simulink model "MSFartoystyring"  (R2013a)
settings: Solver=ode45  StartTime=tstart  StopTime=tstop  RelTol=1e-3
values from neighbouring files (symbols this model uses):
  c = 1    [run.m]
  K_d = (20*xsi*omega_n*T-1)/K    [run.m]
  K_i = 0    [run.m]
  K_i2 = 0.005    [run.m]
  K_p = ((omega_n^2)*T)/K    [run.m]
  K_p2 = 20    [run.m]
  psi0 = 0    [run.m]
  psi_desired = deg2rad(90)    [run.m]
  r0 = 0    [run.m]
  tsamp = 10    [run.m]
  u_desired = 7.3    [run.m]
  v0 = [0.1 0]'    [run.m]
undefined symbols (not defined in the file or in its folder): msfartoystyring
undefined symbols (not defined in the file): p0
settings Model: ExtModeAutoUpdateStatusClock=off  Creator=christh  LastModifiedBy=Mat
settings DataIOCC: SignalLoggingSaveFormat=ModelDataLogs
settings OptimizationCC: ExpressionDepthLimit=2147483647  InitFltsAndDblsToZero=on
settings DebuggingCC: FcnCallInpInsideContextMsg=UseLocalSettings
settings GRTTargetCC: CombineOutputUpdateFcns=off  GRTInterface=on

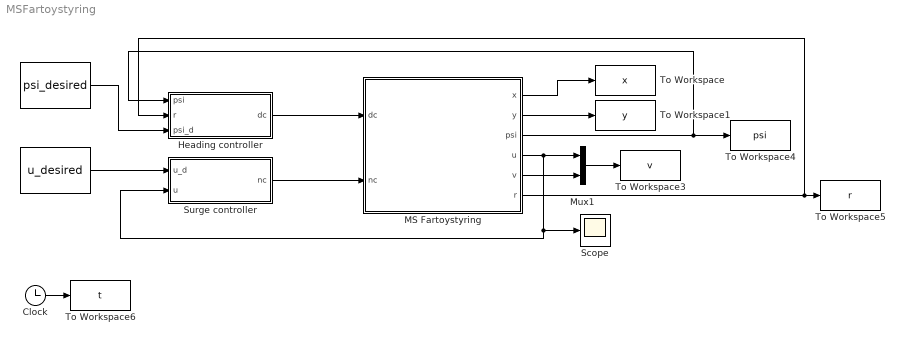
== system MSFartoystyring ==
  " " : Constant  Value=psi_desired
  " " : Constant  Value=u_desired
  Clock : Clock
  Heading controller : Subsystem
  MS Fartoystyring : Subsystem  mask(MS Fartoystyring for Assignment 3 G&C){x0=p0(1), y0=p0(2), u0=v0(1), v0=v0(2), psi0=psi0, r0=r0, c=c}
      mask prompts: x0 "x(t0) (m)"; y0 "y(t0) (m)"; u0 "u(t0) (m/s)"; v0 "v(t0) (m/s)"; psi0 "psi(t0) (rad)"; r0 "r(t0) (rad/s)"; c "current (0 or 1)"
      mask help:
      | Block corresponding to Figure 1 in the assignment text. Gives the response of the ship.
      |
      | The design speed of MS Fartoystyring is u=8.23 m/s.
      |
      | Input:
      | dc: commanded rudder (rad), dmax=25*pi/180
      | nc: commanded shaft speed (rad/s), nmax=85*2*pi/60
      |
      | Output:
      | x: north pos (m)
      | y: east pos (m)
      | u: surge (m/s)
      | v: sway (m/s)
      | psi: heading (rad)
      | r: yaw (rad/s)
      mask Help: Comments, bugs and help requests can be directed to the TA. Email on course website.
  Mux1 : Mux  Inputs=2
  Scope : Scope
  Surge controller : Subsystem
  To Workspace : ToWorkspace  VariableName=x  SampleTime=tsamp
  To Workspace1 : ToWorkspace  VariableName=y  SampleTime=tsamp
  To Workspace3 : ToWorkspace  VariableName=v  SampleTime=tsamp
  To Workspace4 : ToWorkspace  VariableName=psi  SampleTime=tsamp
  To Workspace5 : ToWorkspace  VariableName=r  SampleTime=tsamp
  To Workspace6 : ToWorkspace  VariableName=t  SampleTime=tsamp
  wires:
  Clock/1 -> To Workspace6/1
  MS Fartoystyring/1(x) -> To Workspace/1
  MS Fartoystyring/2(y) -> To Workspace1/1
  MS Fartoystyring/5(v) -> Mux1/2
  Mux1/1 -> To Workspace3/1
  MS Fartoystyring/3(psi) -> To Workspace4/1, Heading controller/1("psi ")
  MS Fartoystyring/6(r) -> Heading controller/2(r), To Workspace5/1
  MS Fartoystyring/4(u) -> Surge controller/2("u "), Scope/1, Mux1/1
  Surge controller/1("nc ") -> MS Fartoystyring/2(nc)
  " "/1 -> Surge controller/1(u_d)
  Heading controller/1("dc ") -> MS Fartoystyring/1(dc)
  " "/1 -> Heading controller/3(psi_d)

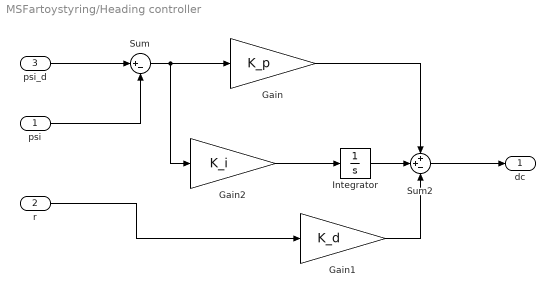
== system MSFartoystyring/Heading controller ==
  "psi " : Inport
  r : Inport  Port=2
  psi_d : Inport  Port=3
  Gain : Gain  Gain=K_p
  Gain1 : Gain  Gain=K_d
  Gain2 : Gain  Gain=K_i
  Integrator : Integrator
  Sum : Sum  Inputs=|+-
  Sum2 : Sum  Inputs=++-
  "dc " : Outport
  wires:
  psi_d/1 -> Sum/1
  "psi "/1 -> Sum/2
  Sum/1 -> Gain2/1, Gain/1
  Gain/1 -> Sum2/1
  Gain2/1 -> Integrator/1
  Integrator/1 -> Sum2/2
  r/1 -> Gain1/1
  Gain1/1 -> Sum2/3
  Sum2/1 -> "dc "/1

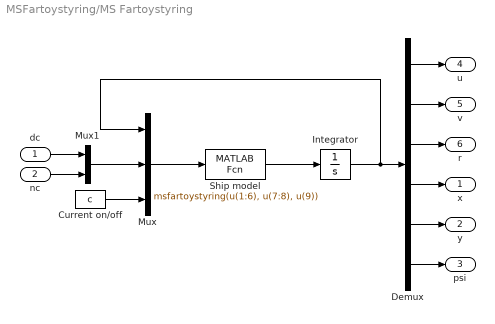
== system MSFartoystyring/MS Fartoystyring ==
  dc : Inport
  nc : Inport  Port=2
  Current on/off : Constant  Value=c
  Demux : Demux  Outputs=6
  Integrator : Integrator  InitialCondition=[u0 v0 r0 x0 y0 psi0]'
  Mux : Mux  Inputs=3
  Mux1 : Mux  Inputs=2
  Ship model : MATLABFcn  MATLABFcn=msfartoystyring(u(1:6), u(7:8), u(9))  OutputDimensions=6
  x : Outport
  y : Outport  Port=2
  psi : Outport  Port=3
  u : Outport  Port=4
  v : Outport  Port=5
  r : Outport  Port=6
  wires:
  Integrator/1 -> Mux/1, Demux/1
  Mux1/1 -> Mux/2
  dc/1 -> Mux1/1
  nc/1 -> Mux1/2
  Demux/1 -> u/1
  Demux/2 -> v/1
  Demux/3 -> r/1
  Demux/4 -> x/1
  Demux/5 -> y/1
  Demux/6 -> psi/1
  Current on/off/1 -> Mux/3
  Ship model/1 -> Integrator/1
  Mux/1 -> Ship model/1

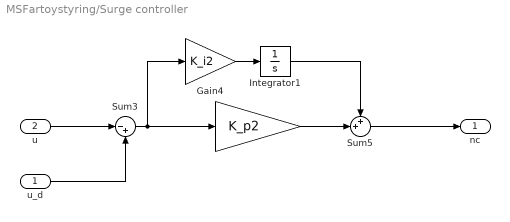
== system MSFartoystyring/Surge controller ==
  u_d : Inport
  "u " : Inport  Port=2
  " " : Gain  Gain=K_p2
  Gain4 : Gain  Gain=K_i2
  Integrator1 : Integrator
  Sum3 : Sum  Inputs=|-+
  Sum5 : Sum  Inputs=++|
  "nc " : Outport
  wires:
  u_d/1 -> Sum3/2
  Sum3/1 -> " "/1, Gain4/1
  Integrator1/1 -> Sum5/1
  " "/1 -> Sum5/2
  Sum5/1 -> "nc "/1
  "u "/1 -> Sum3/1
  Gain4/1 -> Integrator1/1
